simulink library "STLLib"  (R2015a)
settings: Solver=ode45  StartTime=0.0  StopTime=10.0  RelTol=1e-3
libraries: simulink_extras x3
settings Model: Creator=balsi  LastModifiedBy=balsi

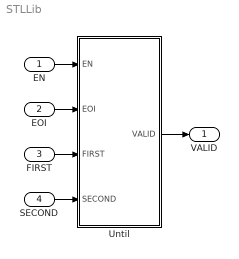
== system STLLib ==
  EN : Inport
  EOI : Inport  Port=2
  FIRST : Inport  Port=3
  SECOND : Inport  Port=4
  Until : Subsystem
  VALID : Outport
  wires:
  EN/1 -> Until/1(EN)
  EOI/1 -> Until/2(EOI)
  SECOND/1 -> Until/4(SECOND)
  Until/1(VALID) -> VALID/1
  FIRST/1 -> Until/3(FIRST)

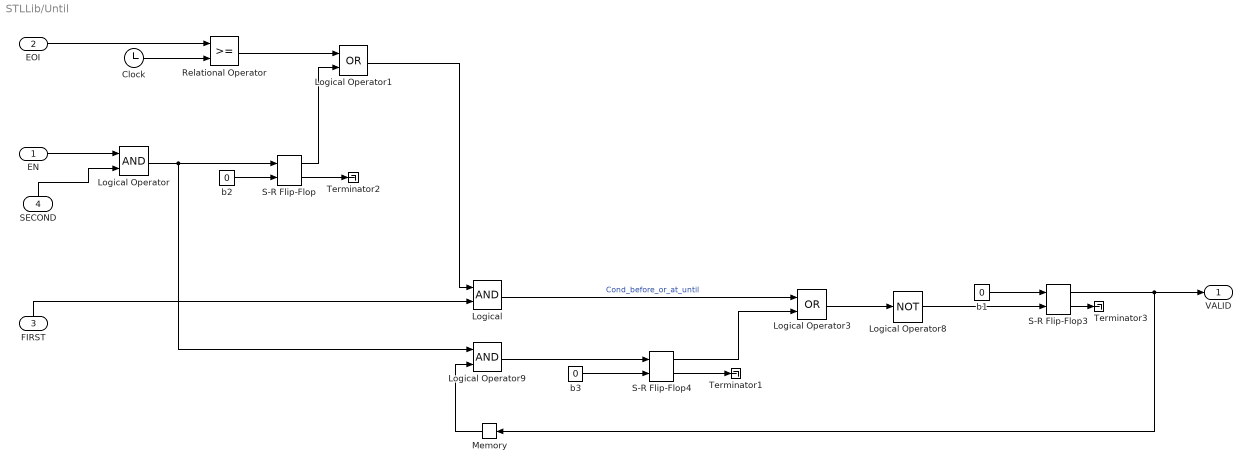
== system STLLib/Until ==
  EN : Inport
  EOI : Inport  Port=2
  FIRST : Inport  Port=3
  SECOND : Inport  Port=4
  Clock : Clock
  "Logical " : Logic  AllPortsSameDT=off  OutDataTypeStr=boolean
  Logical Operator : Logic  AllPortsSameDT=off  OutDataTypeStr=boolean
  Logical Operator1 : Logic  Operator=OR  AllPortsSameDT=off  OutDataTypeStr=boolean
  Logical Operator3 : Logic  Operator=OR  AllPortsSameDT=off  OutDataTypeStr=boolean
  Logical Operator8 : Logic  Operator=NOT  Inputs=1  AllPortsSameDT=off  OutDataTypeStr=boolean
  Logical Operator9 : Logic  AllPortsSameDT=off  OutDataTypeStr=boolean
  Memory : Memory
  Relational Operator : RelationalOperator  OutDataTypeStr=boolean
  S-R Flip-Flop : simulink_extras/Flip Flops/S-R Flip-Flop  initial_condition=0
  S-R Flip-Flop3 : simulink_extras/Flip Flops/S-R Flip-Flop  initial_condition=1
  S-R Flip-Flop4 : simulink_extras/Flip Flops/S-R Flip-Flop  initial_condition=0
  Terminator1 : Terminator
  Terminator2 : Terminator
  Terminator3 : Terminator
  b1 : Constant  Value=0  OutDataTypeStr=boolean
  b2 : Constant  Value=0  OutDataTypeStr=boolean
  b3 : Constant  Value=0  OutDataTypeStr=boolean
  VALID : Outport
  wires:
  S-R Flip-Flop/2 -> Terminator2/1
  "Logical "/1 -> Logical Operator3/1  "Cond_before_or_at_until"
  S-R Flip-Flop4/2 -> Terminator1/1
  Clock/1 -> Relational Operator/2
  b1/1 -> S-R Flip-Flop3/1
  S-R Flip-Flop3/2 -> Terminator3/1
  EN/1 -> Logical Operator/1
  b2/1 -> S-R Flip-Flop/2
  Logical Operator1/1 -> "Logical "/1
  Logical Operator/1 -> S-R Flip-Flop/1, Logical Operator9/1
  S-R Flip-Flop3/1 -> VALID/1, Memory/1
  Relational Operator/1 -> Logical Operator1/1
  Logical Operator3/1 -> Logical Operator8/1
  SECOND/1 -> Logical Operator/2
  FIRST/1 -> "Logical "/2
  Memory/1 -> Logical Operator9/2
  Logical Operator9/1 -> S-R Flip-Flop4/1
  S-R Flip-Flop/1 -> Logical Operator1/2
  S-R Flip-Flop4/1 -> Logical Operator3/2
  Logical Operator8/1 -> S-R Flip-Flop3/2
  EOI/1 -> Relational Operator/1
  b3/1 -> S-R Flip-Flop4/2
